simulink model "Pendulo_doble"  (R2023a)
settings: Solver=VariableStepAuto  StartTime=0.0  StopTime=2  MaxStep=0.01  RelTol=1e-3
values from neighbouring files (symbols this model uses):
  g = 9.81    [Pendulo_parametros.m]
  l1 = 0.3    [Pendulo_parametros.m]
  l2 = 0.25    [Pendulo_parametros.m]
  m1 = 0.2    [Pendulo_parametros.m]
  m2 = 0.1    [Pendulo_parametros.m]
settings Model: Creator=josel
settings OptimizationCC: ReuseModelBlockBuffer=off
settings DebuggingCC: AlgebraicLoopMsg=none

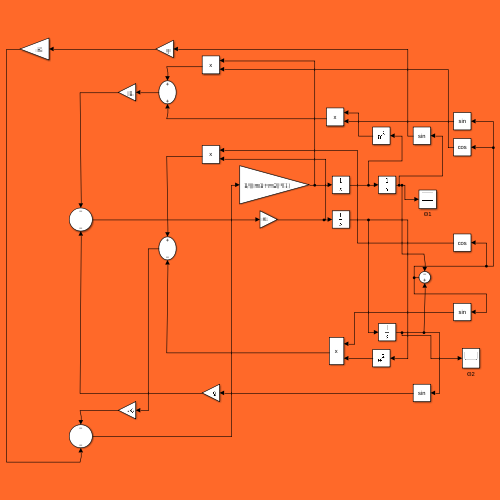
[thumbnail: Simulink's stored preview of the top-level diagram]
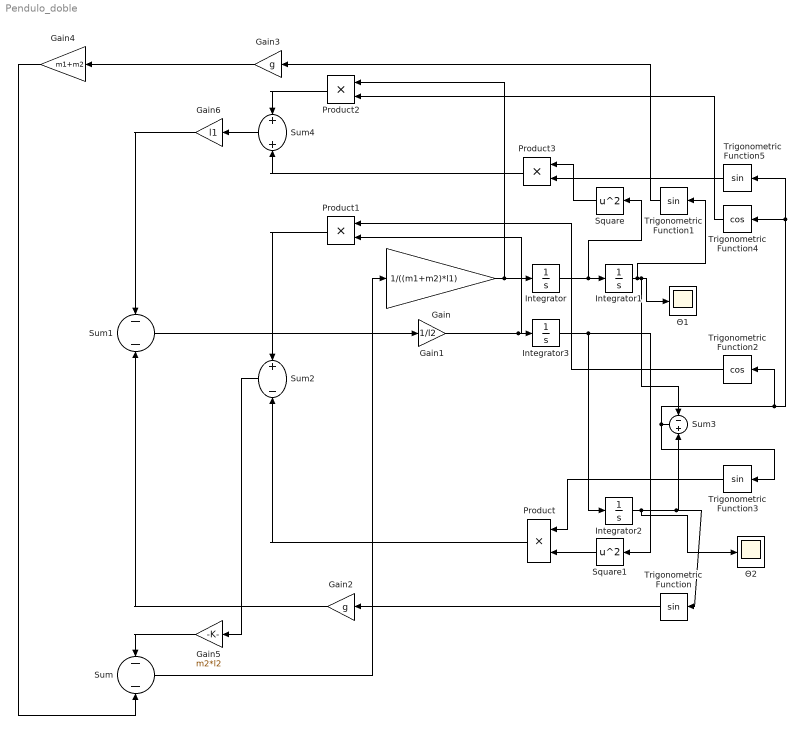
== system Pendulo_doble ==
  Gain : Gain  Gain=1/((m1+m2)*l1)
  Gain1 : Gain  Gain=1/l2
  Gain2 : Gain  Gain=g
  Gain3 : Gain  Gain=g
  Gain4 : Gain  Gain=m1+m2
  Gain5 : Gain  Gain=m2*l2
  Gain6 : Gain  Gain=l1
  Integrator : Integrator
  Integrator1 : Integrator
  Integrator2 : Integrator  InitialCondition=(35*pi)/180
  Integrator3 : Integrator
  Product{,1..3} (4 alike) : Product
  Square : Math  Operator=square
  Square1 : Math  Operator=square
  Sum : Sum  Inputs=--
  Sum1 : Sum  Inputs=--
  Sum2 : Sum  Inputs=+-
  Sum3 : Sum  Inputs=-+
  Sum4 : Sum
  Trigonometric Function{,1,3,5} (4 alike) : Trigonometry
  Trigonometric Function2 : Trigonometry  Operator=cos
  Trigonometric Function4 : Trigonometry  Operator=cos
  Θ1 : Scope
  Θ2 : Scope
  wires:
  Trigonometric Function/1 -> Gain2/1
  Sum3/1 -> Trigonometric Function4/1, Trigonometric Function5/1, Trigonometric Function2/1, Trigonometric Function3/1
  Trigonometric Function4/1 -> Product2/2
  Integrator1/1 -> Θ1/1, Sum3/1, Trigonometric Function1/1
  Square/1 -> Product3/1
  Trigonometric Function1/1 -> Gain3/1
  Integrator3/1 -> Integrator2/1, Square1/1
  Product/1 -> Sum2/2
  Product3/1 -> Sum4/2
  Gain4/1 -> Sum/2
  Trigonometric Function2/1 -> Product1/1
  Square1/1 -> Product/2
  Sum1/1 -> Gain1/1
  Gain1/1 -> Product1/2, Integrator3/1
  Integrator/1 -> Integrator1/1, Square/1
  Sum/1 -> Gain/1
  Gain6/1 -> Sum1/1
  Trigonometric Function5/1 -> Product3/2
  Gain5/1 -> Sum/1
  Product1/1 -> Sum2/1
  Trigonometric Function3/1 -> Product/1
  Gain/1 -> Integrator/1, Product2/1
  Sum4/1 -> Gain6/1
  Integrator2/1 -> Sum3/2, Trigonometric Function/1, Θ2/1
  Sum2/1 -> Gain5/1
  Product2/1 -> Sum4/1
  Gain3/1 -> Gain4/1
  Gain2/1 -> Sum1/2
